simulink model "full_adder"  (R2015a)
settings: Solver=ode23t  StartTime=0.0  StopTime=4  RelTol=1e-3
libraries: fl_lib x281, nesl_utility x271, elec_lib x25
(part 1 of 4)
settings Model: Creator=tomas  LastModifiedBy=tomas

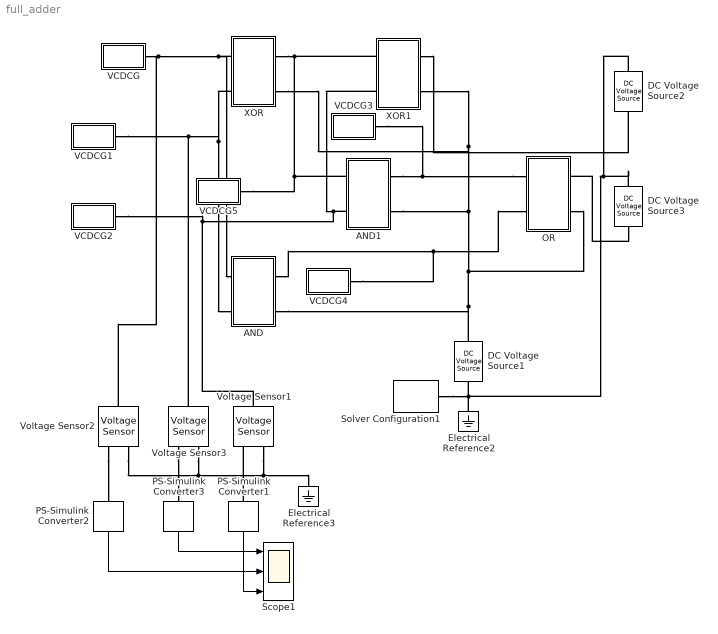
== system full_adder ==
  AND : Subsystem
  AND1 : Subsystem
  DC Voltage Source1 : fl_lib/Electrical/Electrical Sources/DC Voltage Source  v0=1 V
  DC Voltage Source2 : fl_lib/Electrical/Electrical Sources/DC Voltage Source  v0=1 V
  DC Voltage Source3 : fl_lib/Electrical/Electrical Sources/DC Voltage Source  v0=1 V
  Electrical Reference2 : fl_lib/Electrical/Electrical Elements/Electrical Reference
  Electrical Reference3 : fl_lib/Electrical/Electrical Elements/Electrical Reference
  OR : Subsystem
  PS-Simulink Converter1 : nesl_utility/PS-Simulink Converter  PhysicalDomain=network_engine_domain  SubClassName=ps_output  LeftPortType=input  RightPortType=output  PseudoPeriodic=off  Frequencies=[]  Unit=1  AffineConversion=off
  PS-Simulink Converter2 : nesl_utility/PS-Simulink Converter  PhysicalDomain=network_engine_domain  SubClassName=ps_output  LeftPortType=input  RightPortType=output  PseudoPeriodic=off  Frequencies=[]  Unit=1  AffineConversion=off
  PS-Simulink Converter3 : nesl_utility/PS-Simulink Converter  PhysicalDomain=network_engine_domain  SubClassName=ps_output  LeftPortType=input  RightPortType=output  PseudoPeriodic=off  Frequencies=[]  Unit=1  AffineConversion=off
  Scope1 : Scope  NumInputPorts=3
      settings: YMin=-10~-11~-5.5  YMax=0~0~-0.5
  Solver Configuration1 : nesl_utility/Solver Configuration  PhysicalDomain=network_engine_domain  SubClassName=solver  LeftPortType=input  RightPortType=generic  Accelerate=off  Tones=[]  Harmonics=[]  SimulateNoise=off  Profile=off  UseLocalSampling=off  EnableSwitchedLinearOptims=on  FrequencyDomain=off  UseCCode=off  RelTol=0.001  AbsTol=1e-06  MinStep=1e-09  ToWorkspace=off  RevertToSquareIcSolve=off  NumHomotopyIterations=100  DoDC=off  ResidualTolerance=1e-09  UseLocalSolver=off  LocalSolverChoice=NE_BACKWARD_EULER_ADVANCER  LocalSolverSampleTime=0.001  DoFixedCost=off  MaxNonlinIter=3  MaxModeIter=2  LinearAlgebra=Sparse  DelaysMemoryBudget=1024  AutomaticFiltering=on  FilteringTimeConstant=0.001
  VCDCG : Subsystem
  VCDCG1 : Subsystem
  VCDCG2 : Subsystem
  VCDCG3 : Subsystem
  VCDCG4 : Subsystem
  VCDCG5 : Subsystem
  Voltage Sensor1 : fl_lib/Electrical/Electrical Sensors/Voltage Sensor
  Voltage Sensor2 : fl_lib/Electrical/Electrical Sensors/Voltage Sensor
  Voltage Sensor3 : fl_lib/Electrical/Electrical Sensors/Voltage Sensor
  XOR : Subsystem
  XOR1 : Subsystem
  wires:
  PS-Simulink Converter3/1 -> Scope1/1
  PS-Simulink Converter2/1 -> Scope1/2
  PS-Simulink Converter1/1 -> Scope1/3
  connections:
  Electrical Reference2/LConn1 -- DC Voltage Source3/LConn1 -- DC Voltage Source2/LConn1 -- DC Voltage Source1/RConn1 -- Solver Configuration1/RConn1
  DC Voltage Source1/LConn1 -- AND1/RConn2 -- XOR1/RConn2 -- XOR/RConn2 -- OR/RConn2 -- AND/RConn2
  XOR/LConn2 -- VCDCG1/RConn1 -- Voltage Sensor3/LConn1 -- AND/LConn2
  XOR/LConn1 -- Voltage Sensor2/LConn1 -- VCDCG/RConn1 -- AND/LConn1
  XOR/RConn1 -- XOR1/LConn1 -- AND1/LConn1 -- VCDCG5/RConn1
  OR/LConn1 -- AND1/RConn1 -- VCDCG3/RConn1
  AND/RConn1 -- VCDCG4/RConn1 -- OR/LConn2
  VCDCG2/RConn1 -- Voltage Sensor1/LConn1 -- AND1/LConn2 -- XOR1/LConn2
  Voltage Sensor3/RConn2 -- Voltage Sensor2/RConn2 -- Voltage Sensor1/RConn2 -- Electrical Reference3/LConn1
  Voltage Sensor2/RConn1 -- PS-Simulink Converter2/LConn1
  Voltage Sensor3/RConn1 -- PS-Simulink Converter3/LConn1
  PS-Simulink Converter1/LConn1 -- Voltage Sensor1/RConn1
  DC Voltage Source3/RConn1 -- OR/RConn1
  XOR1/RConn1 -- DC Voltage Source2/RConn1

== system full_adder/AND ==
  DCM : Subsystem
  DCM1 : Subsystem
  DCM2 : Subsystem
  Electrical Reference : fl_lib/Electrical/Electrical Elements/Electrical Reference
  Electrical Reference1 : fl_lib/Electrical/Electrical Elements/Electrical Reference
  Out Terminal : Constant  Value=[1 0 0 0; 0 1 0 0; 0 0 1 0; 2 2 -1 -2; -4 -4 7 2]  VectorParams1D=off
  Resistor : elec_lib/Passive Devices/Resistor  R=16 kOhm  noise_mode=0  Tdevice=25 C  sample_time=0.001 s  repeatability=1  auto_seed=1456083514  user_seed=0
  Resistor1 : elec_lib/Passive Devices/Resistor  R=16 kOhm  noise_mode=0  Tdevice=25 C  sample_time=0.001 s  repeatability=1  auto_seed=3847689602  user_seed=0
  Terminal1 : Constant  Value=[0 -1 1 1; 1 0 0 0; 0 0 1 0; 1 0 0 0; 4 1 -3 -1]  VectorParams1D=off
  Terminal2 : Constant  Value=[-1 0 1 1; 0 1 0 0; 0 0 1 0; 0 1 0 0; 1 4 -3 -1]  VectorParams1D=off
  Voltage Sensor{,1..3} (4 alike) : fl_lib/Electrical/Electrical Sensors/Voltage Sensor
  v1 : PMIOPort  Port=1  Side=Left
  v2 : PMIOPort  Port=2  Side=Left
  vo : PMIOPort  Port=3  Side=Right
  vc : PMIOPort  Port=4  Side=Right
  wires:
  Terminal2/1 -> DCM1/1(m)
  Out Terminal/1 -> DCM2/1(m)
  Terminal1/1 -> DCM/1(m)
  connections:
  Voltage Sensor/LConn1 -- DCM/RConn2 -- Resistor/LConn1 -- v1/RConn1
  Voltage Sensor1/LConn1 -- DCM1/RConn2 -- Resistor1/LConn1 -- v2/RConn1
  DCM2/RConn1 -- Voltage Sensor1/RConn1 -- DCM1/RConn1 -- DCM/RConn1
  DCM2/LConn1 -- DCM1/LConn1 -- DCM/LConn1 -- Voltage Sensor/RConn1
  Voltage Sensor2/LConn1 -- DCM2/RConn2 -- Resistor/RConn1 -- Resistor1/RConn1 -- vo/RConn1
  Voltage Sensor2/RConn2 -- Voltage Sensor1/RConn2 -- Electrical Reference/LConn1 -- Voltage Sensor/RConn2
  DCM2/LConn2 -- Voltage Sensor2/RConn1 -- DCM1/LConn2 -- DCM/LConn2
  Voltage Sensor3/LConn1 -- vc/RConn1
  DCM2/LConn3 -- DCM1/LConn3 -- DCM/LConn3 -- Voltage Sensor3/RConn1
  Voltage Sensor3/RConn2 -- Electrical Reference1/LConn1

== system full_adder/AND1 ==
  DCM : Subsystem
  DCM1 : Subsystem
  DCM2 : Subsystem
  Electrical Reference : fl_lib/Electrical/Electrical Elements/Electrical Reference
  Electrical Reference1 : fl_lib/Electrical/Electrical Elements/Electrical Reference
  Out Terminal : Constant  Value=[1 0 0 0; 0 1 0 0; 0 0 1 0; 2 2 -1 -2; -4 -4 7 2]  VectorParams1D=off
  Resistor : elec_lib/Passive Devices/Resistor  R=16 kOhm  noise_mode=0  Tdevice=25 C  sample_time=0.001 s  repeatability=1  auto_seed=1903427766  user_seed=0
  Resistor1 : elec_lib/Passive Devices/Resistor  R=16 kOhm  noise_mode=0  Tdevice=25 C  sample_time=0.001 s  repeatability=1  auto_seed=400135898  user_seed=0
  Terminal1 : Constant  Value=[0 -1 1 1; 1 0 0 0; 0 0 1 0; 1 0 0 0; 4 1 -3 -1]  VectorParams1D=off
  Terminal2 : Constant  Value=[-1 0 1 1; 0 1 0 0; 0 0 1 0; 0 1 0 0; 1 4 -3 -1]  VectorParams1D=off
  Voltage Sensor{,1..3} (4 alike) : fl_lib/Electrical/Electrical Sensors/Voltage Sensor
  v1 : PMIOPort  Port=1  Side=Left
  v2 : PMIOPort  Port=2  Side=Left
  vo : PMIOPort  Port=3  Side=Right
  vc : PMIOPort  Port=4  Side=Right
  wires:
  Terminal2/1 -> DCM1/1(m)
  Out Terminal/1 -> DCM2/1(m)
  Terminal1/1 -> DCM/1(m)
  connections:
  Voltage Sensor/LConn1 -- Resistor/LConn1 -- v1/RConn1 -- DCM/RConn2
  Voltage Sensor1/LConn1 -- Resistor1/LConn1 -- v2/RConn1 -- DCM1/RConn2
  DCM1/RConn1 -- DCM/RConn1 -- Voltage Sensor1/RConn1 -- DCM2/RConn1
  DCM1/LConn1 -- DCM/LConn1 -- Voltage Sensor/RConn1 -- DCM2/LConn1
  Voltage Sensor2/LConn1 -- Resistor/RConn1 -- Resistor1/RConn1 -- vo/RConn1 -- DCM2/RConn2
  Voltage Sensor2/RConn2 -- Voltage Sensor1/RConn2 -- Electrical Reference/LConn1 -- Voltage Sensor/RConn2
  DCM1/LConn2 -- DCM/LConn2 -- Voltage Sensor2/RConn1 -- DCM2/LConn2
  Voltage Sensor3/LConn1 -- vc/RConn1
  DCM1/LConn3 -- DCM/LConn3 -- Voltage Sensor3/RConn1 -- DCM2/LConn3
  Voltage Sensor3/RConn2 -- Electrical Reference1/LConn1

== system full_adder/OR ==
  DCM : Subsystem
  DCM1 : Subsystem
  DCM2 : Subsystem
  Electrical Reference : fl_lib/Electrical/Electrical Elements/Electrical Reference
  Electrical Reference1 : fl_lib/Electrical/Electrical Elements/Electrical Reference
  Out Terminal : Constant  Value=[0 0 1 0; 2 2 -1 2; 1 0 0 0; 0 1 0 0; -4 -4 7 -2]  VectorParams1D=off  SampleTime=-1
  Resistor : elec_lib/Passive Devices/Resistor  R=16 kOhm  noise_mode=0  Tdevice=25 C  sample_time=0.001 s  repeatability=1  auto_seed=2834987259  user_seed=0
  Resistor1 : elec_lib/Passive Devices/Resistor  R=16 kOhm  noise_mode=0  Tdevice=25 C  sample_time=0.001 s  repeatability=1  auto_seed=2963978059  user_seed=0
  Terminal1 : Constant  Value=[0 0 1 0; 1 0 0 0; 0 -1 1 -1; 1 0 0 0; 4 1 -3 1]  VectorParams1D=off  SampleTime=-1
  Terminal2 : Constant  Value=[0 0 1 0; 0 1 0 0; -1 0 1 -1; 0 1 0 0; 1 4 -3 1 ]  VectorParams1D=off  SampleTime=-1
  Voltage Sensor{,1..3} (4 alike) : fl_lib/Electrical/Electrical Sensors/Voltage Sensor
  v1 : PMIOPort  Port=1  Side=Left
  v2 : PMIOPort  Port=2  Side=Left
  vo : PMIOPort  Port=3  Side=Right
  vc : PMIOPort  Port=4  Side=Right
  wires:
  Terminal2/1 -> DCM1/1(m)
  Out Terminal/1 -> DCM2/1(m)
  Terminal1/1 -> DCM/1(m)
  connections:
  Voltage Sensor/LConn1 -- DCM/RConn2 -- Resistor/LConn1 -- v1/RConn1
  Voltage Sensor1/LConn1 -- DCM1/RConn2 -- Resistor1/LConn1 -- v2/RConn1
  DCM2/RConn1 -- Voltage Sensor1/RConn1 -- DCM1/RConn1 -- DCM/RConn1
  DCM2/LConn1 -- DCM1/LConn1 -- DCM/LConn1 -- Voltage Sensor/RConn1
  Voltage Sensor2/LConn1 -- DCM2/RConn2 -- Resistor/RConn1 -- Resistor1/RConn1 -- vo/RConn1
  Voltage Sensor2/RConn2 -- Voltage Sensor1/RConn2 -- Electrical Reference/LConn1 -- Voltage Sensor/RConn2
  Voltage Sensor2/RConn1 -- DCM2/LConn2 -- DCM1/LConn2 -- DCM/LConn2
  Voltage Sensor3/LConn1 -- vc/RConn1
  DCM2/LConn3 -- DCM1/LConn3 -- DCM/LConn3 -- Voltage Sensor3/RConn1
  Voltage Sensor3/RConn2 -- Electrical Reference1/LConn1

== system full_adder/VCDCG ==
  Controlled Current Source : fl_lib/Electrical/Electrical Sources/Controlled Current Source
  Electrical Reference1 : fl_lib/Electrical/Electrical Elements/Electrical Reference
  Integrator : Integrator  InitialCondition=.001*rand()-.005  LimitOutput=on  UpperSaturationLimit=.2  LowerSaturationLimit=-.2
  MATLAB Function : MATLAB Function  TreatAsAtomicUnit=on
  PS-Simulink Converter : nesl_utility/PS-Simulink Converter  PhysicalDomain=network_engine_domain  SubClassName=ps_output  LeftPortType=input  RightPortType=output  PseudoPeriodic=off  Frequencies=[]  Unit=1  AffineConversion=off
  Simulink-PS Converter : nesl_utility/Simulink-PS Converter  PhysicalDomain=network_engine_domain  SubClassName=ps_input  LeftPortType=input  RightPortType=output  PseudoPeriodic=off  Frequencies=[]  NoiseDistribution=none  NoiseParameters=[]  Unit=1  AffineConversion=off  InputFiltering=off  SimscapeFilterOrder=1  InputFilterTimeConstant=0.001  UdotUserProvided=1
  Voltage Sensor : fl_lib/Electrical/Electrical Sensors/Voltage Sensor
  Out : PMIOPort  Port=1  Side=Right
  wires:
  Integrator/1 -> Simulink-PS Converter/1
  MATLAB Function/1(y) -> Integrator/1
  PS-Simulink Converter/1 -> MATLAB Function/1(u)
  connections:
  Voltage Sensor/RConn2 -- Controlled Current Source/RConn2 -- Electrical Reference1/LConn1
  Voltage Sensor/LConn1 -- Controlled Current Source/LConn1 -- Out/RConn1
  Voltage Sensor/RConn1 -- PS-Simulink Converter/LConn1
  Simulink-PS Converter/RConn1 -- Controlled Current Source/RConn1

== system full_adder/VCDCG1 ==
  Controlled Current Source : fl_lib/Electrical/Electrical Sources/Controlled Current Source
  Electrical Reference1 : fl_lib/Electrical/Electrical Elements/Electrical Reference
  Integrator : Integrator  InitialCondition=.001*rand()-.005  LimitOutput=on  UpperSaturationLimit=.2  LowerSaturationLimit=-.2
  MATLAB Function : MATLAB Function  TreatAsAtomicUnit=on
  PS-Simulink Converter : nesl_utility/PS-Simulink Converter  PhysicalDomain=network_engine_domain  SubClassName=ps_output  LeftPortType=input  RightPortType=output  PseudoPeriodic=off  Frequencies=[]  Unit=1  AffineConversion=off
  Simulink-PS Converter : nesl_utility/Simulink-PS Converter  PhysicalDomain=network_engine_domain  SubClassName=ps_input  LeftPortType=input  RightPortType=output  PseudoPeriodic=off  Frequencies=[]  NoiseDistribution=none  NoiseParameters=[]  Unit=1  AffineConversion=off  InputFiltering=off  SimscapeFilterOrder=1  InputFilterTimeConstant=0.001  UdotUserProvided=1
  Voltage Sensor : fl_lib/Electrical/Electrical Sensors/Voltage Sensor
  Out : PMIOPort  Port=1  Side=Right
  wires:
  Integrator/1 -> Simulink-PS Converter/1
  MATLAB Function/1(y) -> Integrator/1
  PS-Simulink Converter/1 -> MATLAB Function/1(u)
  connections:
  Electrical Reference1/LConn1 -- Voltage Sensor/RConn2 -- Controlled Current Source/RConn2
  Out/RConn1 -- Voltage Sensor/LConn1 -- Controlled Current Source/LConn1
  Voltage Sensor/RConn1 -- PS-Simulink Converter/LConn1
  Simulink-PS Converter/RConn1 -- Controlled Current Source/RConn1

== system full_adder/VCDCG2 ==
  Controlled Current Source : fl_lib/Electrical/Electrical Sources/Controlled Current Source
  Electrical Reference1 : fl_lib/Electrical/Electrical Elements/Electrical Reference
  Integrator : Integrator  InitialCondition=.001*rand()-.005  LimitOutput=on  UpperSaturationLimit=.2  LowerSaturationLimit=-.2
  MATLAB Function : MATLAB Function  TreatAsAtomicUnit=on
  PS-Simulink Converter : nesl_utility/PS-Simulink Converter  PhysicalDomain=network_engine_domain  SubClassName=ps_output  LeftPortType=input  RightPortType=output  PseudoPeriodic=off  Frequencies=[]  Unit=1  AffineConversion=off
  Simulink-PS Converter : nesl_utility/Simulink-PS Converter  PhysicalDomain=network_engine_domain  SubClassName=ps_input  LeftPortType=input  RightPortType=output  PseudoPeriodic=off  Frequencies=[]  NoiseDistribution=none  NoiseParameters=[]  Unit=1  AffineConversion=off  InputFiltering=off  SimscapeFilterOrder=1  InputFilterTimeConstant=0.001  UdotUserProvided=1
  Voltage Sensor : fl_lib/Electrical/Electrical Sensors/Voltage Sensor
  Out : PMIOPort  Port=1  Side=Right
  wires:
  Integrator/1 -> Simulink-PS Converter/1
  MATLAB Function/1(y) -> Integrator/1
  PS-Simulink Converter/1 -> MATLAB Function/1(u)
  connections:
  Electrical Reference1/LConn1 -- Voltage Sensor/RConn2 -- Controlled Current Source/RConn2
  Out/RConn1 -- Voltage Sensor/LConn1 -- Controlled Current Source/LConn1
  Voltage Sensor/RConn1 -- PS-Simulink Converter/LConn1
  Simulink-PS Converter/RConn1 -- Controlled Current Source/RConn1

== system full_adder/VCDCG3 ==
  Controlled Current Source : fl_lib/Electrical/Electrical Sources/Controlled Current Source
  Electrical Reference1 : fl_lib/Electrical/Electrical Elements/Electrical Reference
  Integrator : Integrator  InitialCondition=.001*rand()-.005  LimitOutput=on  UpperSaturationLimit=.2  LowerSaturationLimit=-.2
  MATLAB Function : MATLAB Function  TreatAsAtomicUnit=on
  PS-Simulink Converter : nesl_utility/PS-Simulink Converter  PhysicalDomain=network_engine_domain  SubClassName=ps_output  LeftPortType=input  RightPortType=output  PseudoPeriodic=off  Frequencies=[]  Unit=1  AffineConversion=off
  Simulink-PS Converter : nesl_utility/Simulink-PS Converter  PhysicalDomain=network_engine_domain  SubClassName=ps_input  LeftPortType=input  RightPortType=output  PseudoPeriodic=off  Frequencies=[]  NoiseDistribution=none  NoiseParameters=[]  Unit=1  AffineConversion=off  InputFiltering=off  SimscapeFilterOrder=1  InputFilterTimeConstant=0.001  UdotUserProvided=1
  Voltage Sensor : fl_lib/Electrical/Electrical Sensors/Voltage Sensor
  Out : PMIOPort  Port=1  Side=Right
  wires:
  Integrator/1 -> Simulink-PS Converter/1
  MATLAB Function/1(y) -> Integrator/1
  PS-Simulink Converter/1 -> MATLAB Function/1(u)
  connections:
  Electrical Reference1/LConn1 -- Voltage Sensor/RConn2 -- Controlled Current Source/RConn2
  Out/RConn1 -- Voltage Sensor/LConn1 -- Controlled Current Source/LConn1
  Voltage Sensor/RConn1 -- PS-Simulink Converter/LConn1
  Simulink-PS Converter/RConn1 -- Controlled Current Source/RConn1

== system full_adder/VCDCG4 ==
  Controlled Current Source : fl_lib/Electrical/Electrical Sources/Controlled Current Source
  Electrical Reference1 : fl_lib/Electrical/Electrical Elements/Electrical Reference
  Integrator : Integrator  InitialCondition=.001*rand()-.005  LimitOutput=on  UpperSaturationLimit=.2  LowerSaturationLimit=-.2
  MATLAB Function : MATLAB Function  TreatAsAtomicUnit=on
  PS-Simulink Converter : nesl_utility/PS-Simulink Converter  PhysicalDomain=network_engine_domain  SubClassName=ps_output  LeftPortType=input  RightPortType=output  PseudoPeriodic=off  Frequencies=[]  Unit=1  AffineConversion=off
  Simulink-PS Converter : nesl_utility/Simulink-PS Converter  PhysicalDomain=network_engine_domain  SubClassName=ps_input  LeftPortType=input  RightPortType=output  PseudoPeriodic=off  Frequencies=[]  NoiseDistribution=none  NoiseParameters=[]  Unit=1  AffineConversion=off  InputFiltering=off  SimscapeFilterOrder=1  InputFilterTimeConstant=0.001  UdotUserProvided=1
  Voltage Sensor : fl_lib/Electrical/Electrical Sensors/Voltage Sensor
  Out : PMIOPort  Port=1  Side=Right
  wires:
  Integrator/1 -> Simulink-PS Converter/1
  MATLAB Function/1(y) -> Integrator/1
  PS-Simulink Converter/1 -> MATLAB Function/1(u)
  connections:
  Electrical Reference1/LConn1 -- Voltage Sensor/RConn2 -- Controlled Current Source/RConn2
  Out/RConn1 -- Voltage Sensor/LConn1 -- Controlled Current Source/LConn1
  Voltage Sensor/RConn1 -- PS-Simulink Converter/LConn1
  Simulink-PS Converter/RConn1 -- Controlled Current Source/RConn1

== system full_adder/VCDCG5 ==
  Controlled Current Source : fl_lib/Electrical/Electrical Sources/Controlled Current Source
  Electrical Reference1 : fl_lib/Electrical/Electrical Elements/Electrical Reference
  Integrator : Integrator  InitialCondition=.001*rand()-.005  LimitOutput=on  UpperSaturationLimit=.2  LowerSaturationLimit=-.2
  MATLAB Function : MATLAB Function  TreatAsAtomicUnit=on
  PS-Simulink Converter : nesl_utility/PS-Simulink Converter  PhysicalDomain=network_engine_domain  SubClassName=ps_output  LeftPortType=input  RightPortType=output  PseudoPeriodic=off  Frequencies=[]  Unit=1  AffineConversion=off
  Simulink-PS Converter : nesl_utility/Simulink-PS Converter  PhysicalDomain=network_engine_domain  SubClassName=ps_input  LeftPortType=input  RightPortType=output  PseudoPeriodic=off  Frequencies=[]  NoiseDistribution=none  NoiseParameters=[]  Unit=1  AffineConversion=off  InputFiltering=off  SimscapeFilterOrder=1  InputFilterTimeConstant=0.001  UdotUserProvided=1
  Voltage Sensor : fl_lib/Electrical/Electrical Sensors/Voltage Sensor
  Out : PMIOPort  Port=1  Side=Right
  wires:
  Integrator/1 -> Simulink-PS Converter/1
  MATLAB Function/1(y) -> Integrator/1
  PS-Simulink Converter/1 -> MATLAB Function/1(u)
  connections:
  Electrical Reference1/LConn1 -- Voltage Sensor/RConn2 -- Controlled Current Source/RConn2
  Out/RConn1 -- Voltage Sensor/LConn1 -- Controlled Current Source/LConn1
  Voltage Sensor/RConn1 -- PS-Simulink Converter/LConn1
  Simulink-PS Converter/RConn1 -- Controlled Current Source/RConn1

== system full_adder/XOR ==
  DCM : Subsystem
  DCM1 : Subsystem
  DCM2 : Subsystem
  Electrical Reference : fl_lib/Electrical/Electrical Elements/Electrical Reference
  Electrical Reference1 : fl_lib/Electrical/Electrical Elements/Electrical Reference
  Out Terminal : Constant  Value=[-1 -1 0 1; 1 1 0 1; -1 1 0 -1; 1 -1 0 -1; -1 -1 7 0]  VectorParams1D=off
  Resistor : elec_lib/Passive Devices/Resistor  R=26 kOhm  noise_mode=0  Tdevice=25 C  sample_time=0.001 s  repeatability=1  auto_seed=3482499289  user_seed=0
  Resistor1 : elec_lib/Passive Devices/Resistor  R=26 kOhm  noise_mode=0  Tdevice=25 C  sample_time=0.001 s  repeatability=1  auto_seed=3989505789  user_seed=0
  Terminal1 : Constant  Value=[0 -1 -1 1; 0 1 1 1; 0 -1 1 -1; 0 1 -1 -1; 6 0 -1 0]  VectorParams1D=off
  Terminal2 : Constant  Value=[-1 0 -1 1; 1 0 1 1; -1 0 1 -1; 1 0 -1 -1; 0 6 -1 0]  VectorParams1D=off
  Voltage Sensor{,1..3} (4 alike) : fl_lib/Electrical/Electrical Sensors/Voltage Sensor
  v1 : PMIOPort  Port=1  Side=Left
  v2 : PMIOPort  Port=2  Side=Left
  vo : PMIOPort  Port=3  Side=Right
  vc : PMIOPort  Port=4  Side=Right
  wires:
  Terminal2/1 -> DCM1/1(m)
  Out Terminal/1 -> DCM2/1(m)
  Terminal1/1 -> DCM/1(m)
  connections:
  DCM/RConn2 -- Voltage Sensor/LConn1 -- Resistor/LConn1 -- v1/RConn1
  Voltage Sensor1/LConn1 -- DCM1/RConn2 -- Resistor1/LConn1 -- v2/RConn1
  DCM2/RConn1 -- Voltage Sensor1/RConn1 -- DCM1/RConn1 -- DCM/RConn1
  DCM2/LConn1 -- DCM1/LConn1 -- DCM/LConn1 -- Voltage Sensor/RConn1
  Voltage Sensor2/LConn1 -- DCM2/RConn2 -- Resistor/RConn1 -- Resistor1/RConn1 -- vo/RConn1
  Voltage Sensor2/RConn2 -- Voltage Sensor1/RConn2 -- Electrical Reference/LConn1 -- Voltage Sensor/RConn2
  DCM2/LConn2 -- Voltage Sensor2/RConn1 -- DCM1/LConn2 -- DCM/LConn2
  Voltage Sensor3/LConn1 -- vc/RConn1
  DCM2/LConn3 -- DCM1/LConn3 -- DCM/LConn3 -- Voltage Sensor3/RConn1
  Voltage Sensor3/RConn2 -- Electrical Reference1/LConn1

== system full_adder/XOR1 ==
  DCM : Subsystem
  DCM1 : Subsystem
  DCM2 : Subsystem
  Electrical Reference : fl_lib/Electrical/Electrical Elements/Electrical Reference
  Electrical Reference1 : fl_lib/Electrical/Electrical Elements/Electrical Reference
  Out Terminal : Constant  Value=[-1 -1 0 1; 1 1 0 1; -1 1 0 -1; 1 -1 0 -1; -1 -1 7 0]  VectorParams1D=off
  Resistor : elec_lib/Passive Devices/Resistor  R=26 kOhm  noise_mode=0  Tdevice=25 C  sample_time=0.001 s  repeatability=1  auto_seed=311627844  user_seed=0
  Resistor1 : elec_lib/Passive Devices/Resistor  R=26 kOhm  noise_mode=0  Tdevice=25 C  sample_time=0.001 s  repeatability=1  auto_seed=2729173630  user_seed=0
  Terminal1 : Constant  Value=[0 -1 -1 1; 0 1 1 1; 0 -1 1 -1; 0 1 -1 -1; 6 0 -1 0]  VectorParams1D=off
  Terminal2 : Constant  Value=[-1 0 -1 1; 1 0 1 1; -1 0 1 -1; 1 0 -1 -1; 0 6 -1 0]  VectorParams1D=off
  Voltage Sensor{,1..3} (4 alike) : fl_lib/Electrical/Electrical Sensors/Voltage Sensor
  v1 : PMIOPort  Port=1  Side=Left
  v2 : PMIOPort  Port=2  Side=Left
  vo : PMIOPort  Port=3  Side=Right
  vc : PMIOPort  Port=4  Side=Right
  wires:
  Terminal2/1 -> DCM1/1(m)
  Out Terminal/1 -> DCM2/1(m)
  Terminal1/1 -> DCM/1(m)
  connections:
  DCM/RConn2 -- Voltage Sensor/LConn1 -- Resistor/LConn1 -- v1/RConn1
  Voltage Sensor1/LConn1 -- Resistor1/LConn1 -- v2/RConn1 -- DCM1/RConn2
  DCM1/RConn1 -- DCM/RConn1 -- Voltage Sensor1/RConn1 -- DCM2/RConn1
  DCM1/LConn1 -- DCM/LConn1 -- Voltage Sensor/RConn1 -- DCM2/LConn1
  Voltage Sensor2/LConn1 -- Resistor/RConn1 -- Resistor1/RConn1 -- vo/RConn1 -- DCM2/RConn2
  Voltage Sensor2/RConn2 -- Voltage Sensor1/RConn2 -- Electrical Reference/LConn1 -- Voltage Sensor/RConn2
  DCM1/LConn2 -- DCM/LConn2 -- Voltage Sensor2/RConn1 -- DCM2/LConn2
  Voltage Sensor3/LConn1 -- vc/RConn1
  DCM1/LConn3 -- DCM/LConn3 -- Voltage Sensor3/RConn1 -- DCM2/LConn3
  Voltage Sensor3/RConn2 -- Electrical Reference1/LConn1

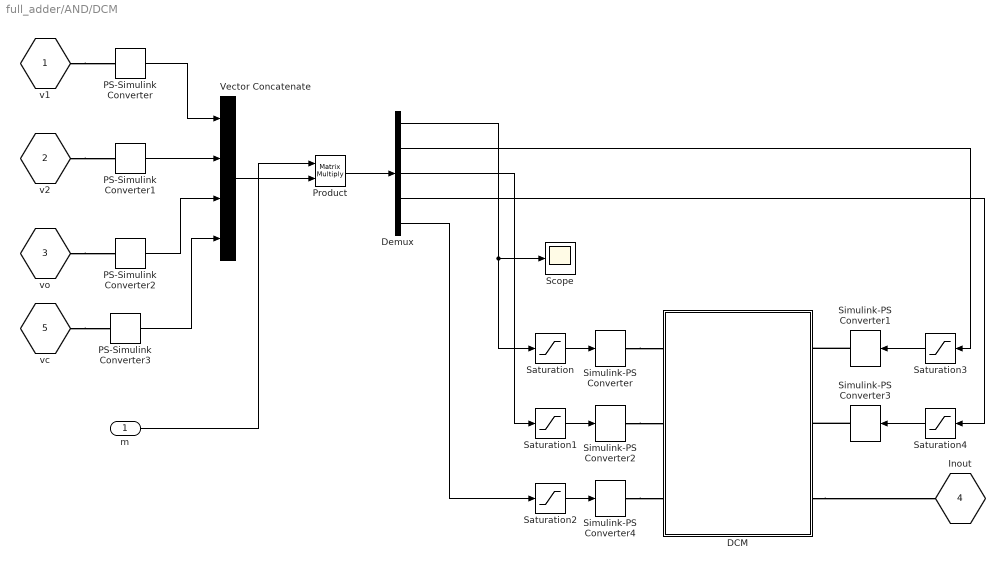
== system full_adder/AND/DCM ==
  m : Inport
  DCM : Subsystem
  Demux : Demux  Outputs=5
  PS-Simulink Converter{,1..3} (4 alike) : nesl_utility/PS-Simulink Converter  PhysicalDomain=network_engine_domain  SubClassName=ps_output  LeftPortType=input  RightPortType=output  PseudoPeriodic=off  Frequencies=[]  Unit=V  AffineConversion=off
  Product : Product  Multiplication=Matrix(*)
  Saturation{,1..4} (5 alike) : Saturate  UpperLimit=10  LowerLimit=-10
  Scope : Scope
      settings: YMin=-30  YMax=15  SaveName=ScopeData3
  Simulink-PS Converter{,1..4} (5 alike) : nesl_utility/Simulink-PS Converter  PhysicalDomain=network_engine_domain  SubClassName=ps_input  LeftPortType=input  RightPortType=output  PseudoPeriodic=off  Frequencies=[]  NoiseDistribution=none  NoiseParameters=[]  Unit=V  AffineConversion=off  InputFiltering=off  SimscapeFilterOrder=1  InputFilterTimeConstant=0.001  UdotUserProvided=1
  Vector Concatenate : Concatenate  NumInputs=4
  "v1 " : PMIOPort  Port=1  Side=Left
  v2 : PMIOPort  Port=2  Side=Right
  vo : PMIOPort  Port=3  Side=Left
  Inout : PMIOPort  Port=4  Side=Right
  vc : PMIOPort  Port=5  Side=Left
  wires:
  PS-Simulink Converter3/1 -> Vector Concatenate/4
  PS-Simulink Converter/1 -> Vector Concatenate/1
  PS-Simulink Converter2/1 -> Vector Concatenate/3
  PS-Simulink Converter1/1 -> Vector Concatenate/2
  Demux/1 -> Scope/1, Saturation/1
  m/1 -> Product/1
  Vector Concatenate/1 -> Product/2
  Product/1 -> Demux/1
  Saturation/1 -> Simulink-PS Converter/1
  Demux/3 -> Saturation1/1
  Saturation1/1 -> Simulink-PS Converter2/1
  Demux/5 -> Saturation2/1
  Saturation2/1 -> Simulink-PS Converter4/1
  Saturation3/1 -> Simulink-PS Converter1/1
  Demux/2 -> Saturation3/1
  Saturation4/1 -> Simulink-PS Converter3/1
  Demux/4 -> Saturation4/1
  connections:
  Simulink-PS Converter2/RConn1 -- DCM/LConn2
  DCM/RConn3 -- Inout/RConn1
  Simulink-PS Converter3/RConn1 -- DCM/RConn2
  vo/RConn1 -- PS-Simulink Converter2/LConn1
  Simulink-PS Converter4/RConn1 -- DCM/LConn3
  Simulink-PS Converter/RConn1 -- DCM/LConn1
  "v1 "/RConn1 -- PS-Simulink Converter/LConn1
  v2/RConn1 -- PS-Simulink Converter1/LConn1
  Simulink-PS Converter1/RConn1 -- DCM/RConn1
  vc/RConn1 -- PS-Simulink Converter3/LConn1

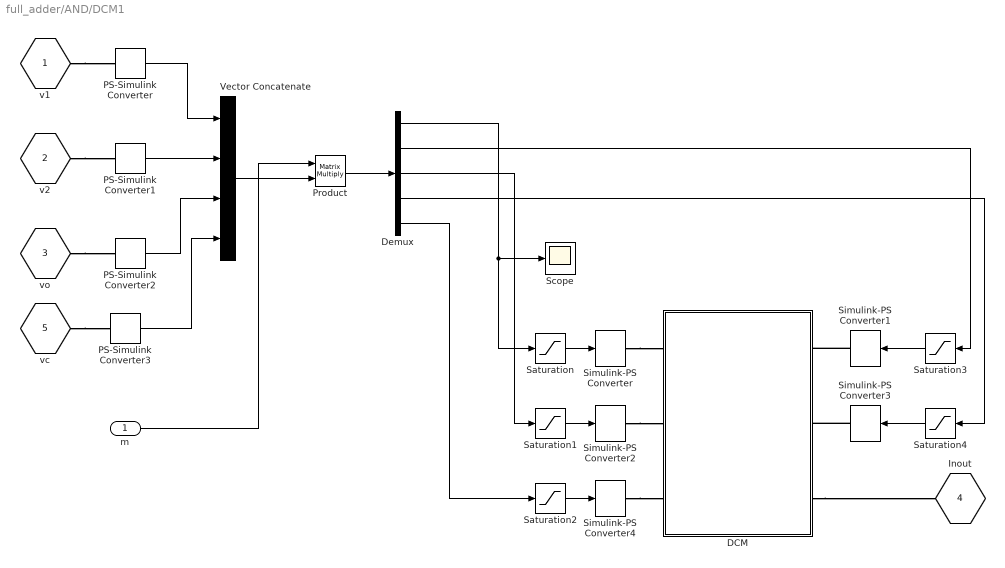
== system full_adder/AND/DCM1 ==
  m : Inport
  DCM : Subsystem
  Demux : Demux  Outputs=5
  PS-Simulink Converter{,1..3} (4 alike) : nesl_utility/PS-Simulink Converter  PhysicalDomain=network_engine_domain  SubClassName=ps_output  LeftPortType=input  RightPortType=output  PseudoPeriodic=off  Frequencies=[]  Unit=V  AffineConversion=off
  Product : Product  Multiplication=Matrix(*)
  Saturation{,1..4} (5 alike) : Saturate  UpperLimit=10  LowerLimit=-10
  Scope : Scope
      settings: YMin=-30  YMax=15  SaveName=ScopeData3
  Simulink-PS Converter{,1..4} (5 alike) : nesl_utility/Simulink-PS Converter  PhysicalDomain=network_engine_domain  SubClassName=ps_input  LeftPortType=input  RightPortType=output  PseudoPeriodic=off  Frequencies=[]  NoiseDistribution=none  NoiseParameters=[]  Unit=V  AffineConversion=off  InputFiltering=off  SimscapeFilterOrder=1  InputFilterTimeConstant=0.001  UdotUserProvided=1
  Vector Concatenate : Concatenate  NumInputs=4
  "v1 " : PMIOPort  Port=1  Side=Left
  v2 : PMIOPort  Port=2  Side=Right
  vo : PMIOPort  Port=3  Side=Left
  Inout : PMIOPort  Port=4  Side=Right
  vc : PMIOPort  Port=5  Side=Left
  wires:
  PS-Simulink Converter3/1 -> Vector Concatenate/4
  PS-Simulink Converter/1 -> Vector Concatenate/1
  PS-Simulink Converter2/1 -> Vector Concatenate/3
  PS-Simulink Converter1/1 -> Vector Concatenate/2
  Demux/1 -> Scope/1, Saturation/1
  m/1 -> Product/1
  Vector Concatenate/1 -> Product/2
  Product/1 -> Demux/1
  Saturation/1 -> Simulink-PS Converter/1
  Demux/3 -> Saturation1/1
  Saturation1/1 -> Simulink-PS Converter2/1
  Demux/5 -> Saturation2/1
  Saturation2/1 -> Simulink-PS Converter4/1
  Saturation3/1 -> Simulink-PS Converter1/1
  Demux/2 -> Saturation3/1
  Saturation4/1 -> Simulink-PS Converter3/1
  Demux/4 -> Saturation4/1
  connections:
  Simulink-PS Converter2/RConn1 -- DCM/LConn2
  DCM/RConn3 -- Inout/RConn1
  Simulink-PS Converter3/RConn1 -- DCM/RConn2
  vo/RConn1 -- PS-Simulink Converter2/LConn1
  Simulink-PS Converter4/RConn1 -- DCM/LConn3
  Simulink-PS Converter/RConn1 -- DCM/LConn1
  "v1 "/RConn1 -- PS-Simulink Converter/LConn1
  v2/RConn1 -- PS-Simulink Converter1/LConn1
  Simulink-PS Converter1/RConn1 -- DCM/RConn1
  vc/RConn1 -- PS-Simulink Converter3/LConn1

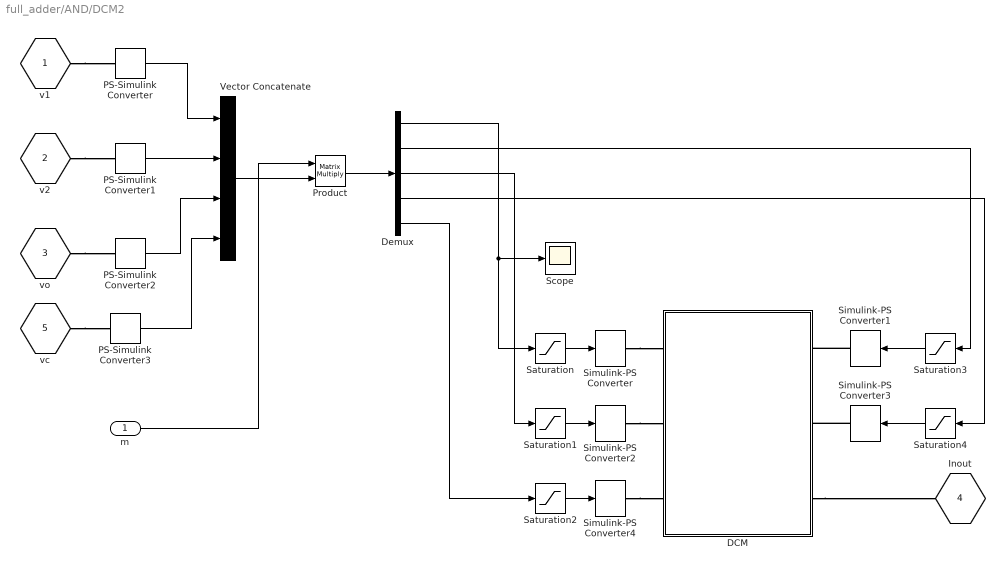
== system full_adder/AND/DCM2 ==
  m : Inport
  DCM : Subsystem
  Demux : Demux  Outputs=5
  PS-Simulink Converter{,1..3} (4 alike) : nesl_utility/PS-Simulink Converter  PhysicalDomain=network_engine_domain  SubClassName=ps_output  LeftPortType=input  RightPortType=output  PseudoPeriodic=off  Frequencies=[]  Unit=V  AffineConversion=off
  Product : Product  Multiplication=Matrix(*)
  Saturation{,1..4} (5 alike) : Saturate  UpperLimit=10  LowerLimit=-10
  Scope : Scope
      settings: YMin=-30  YMax=15  SaveName=ScopeData3
  Simulink-PS Converter{,1..4} (5 alike) : nesl_utility/Simulink-PS Converter  PhysicalDomain=network_engine_domain  SubClassName=ps_input  LeftPortType=input  RightPortType=output  PseudoPeriodic=off  Frequencies=[]  NoiseDistribution=none  NoiseParameters=[]  Unit=V  AffineConversion=off  InputFiltering=off  SimscapeFilterOrder=1  InputFilterTimeConstant=0.001  UdotUserProvided=1
  Vector Concatenate : Concatenate  NumInputs=4
  "v1 " : PMIOPort  Port=1  Side=Left
  v2 : PMIOPort  Port=2  Side=Right
  vo : PMIOPort  Port=3  Side=Left
  Inout : PMIOPort  Port=4  Side=Right
  vc : PMIOPort  Port=5  Side=Left
  wires:
  PS-Simulink Converter3/1 -> Vector Concatenate/4
  PS-Simulink Converter/1 -> Vector Concatenate/1
  PS-Simulink Converter2/1 -> Vector Concatenate/3
  PS-Simulink Converter1/1 -> Vector Concatenate/2
  Demux/1 -> Scope/1, Saturation/1
  m/1 -> Product/1
  Vector Concatenate/1 -> Product/2
  Product/1 -> Demux/1
  Saturation/1 -> Simulink-PS Converter/1
  Demux/3 -> Saturation1/1
  Saturation1/1 -> Simulink-PS Converter2/1
  Demux/5 -> Saturation2/1
  Saturation2/1 -> Simulink-PS Converter4/1
  Saturation3/1 -> Simulink-PS Converter1/1
  Demux/2 -> Saturation3/1
  Saturation4/1 -> Simulink-PS Converter3/1
  Demux/4 -> Saturation4/1
  connections:
  Simulink-PS Converter2/RConn1 -- DCM/LConn2
  DCM/RConn3 -- Inout/RConn1
  Simulink-PS Converter3/RConn1 -- DCM/RConn2
  vo/RConn1 -- PS-Simulink Converter2/LConn1
  Simulink-PS Converter4/RConn1 -- DCM/LConn3
  Simulink-PS Converter/RConn1 -- DCM/LConn1
  "v1 "/RConn1 -- PS-Simulink Converter/LConn1
  v2/RConn1 -- PS-Simulink Converter1/LConn1
  Simulink-PS Converter1/RConn1 -- DCM/RConn1
  vc/RConn1 -- PS-Simulink Converter3/LConn1

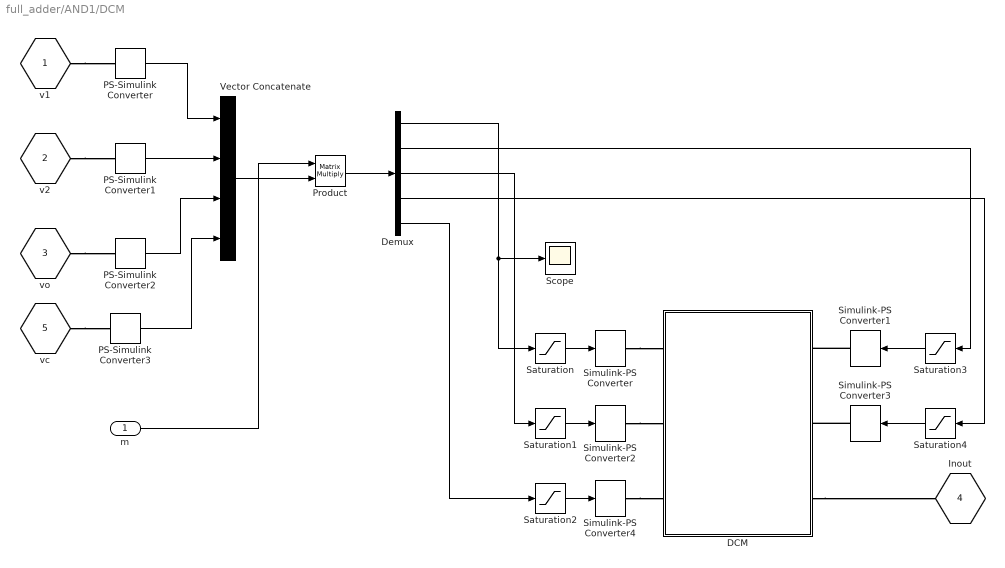
== system full_adder/AND1/DCM ==
  m : Inport
  DCM : Subsystem
  Demux : Demux  Outputs=5
  PS-Simulink Converter{,1..3} (4 alike) : nesl_utility/PS-Simulink Converter  PhysicalDomain=network_engine_domain  SubClassName=ps_output  LeftPortType=input  RightPortType=output  PseudoPeriodic=off  Frequencies=[]  Unit=V  AffineConversion=off
  Product : Product  Multiplication=Matrix(*)
  Saturation{,1..4} (5 alike) : Saturate  UpperLimit=10  LowerLimit=-10
  Scope : Scope
      settings: YMin=-30  YMax=15  SaveName=ScopeData3
  Simulink-PS Converter{,1..4} (5 alike) : nesl_utility/Simulink-PS Converter  PhysicalDomain=network_engine_domain  SubClassName=ps_input  LeftPortType=input  RightPortType=output  PseudoPeriodic=off  Frequencies=[]  NoiseDistribution=none  NoiseParameters=[]  Unit=V  AffineConversion=off  InputFiltering=off  SimscapeFilterOrder=1  InputFilterTimeConstant=0.001  UdotUserProvided=1
  Vector Concatenate : Concatenate  NumInputs=4
  "v1 " : PMIOPort  Port=1  Side=Left
  v2 : PMIOPort  Port=2  Side=Right
  vo : PMIOPort  Port=3  Side=Left
  Inout : PMIOPort  Port=4  Side=Right
  vc : PMIOPort  Port=5  Side=Left
  wires:
  PS-Simulink Converter3/1 -> Vector Concatenate/4
  PS-Simulink Converter/1 -> Vector Concatenate/1
  PS-Simulink Converter2/1 -> Vector Concatenate/3
  PS-Simulink Converter1/1 -> Vector Concatenate/2
  Demux/1 -> Scope/1, Saturation/1
  m/1 -> Product/1
  Vector Concatenate/1 -> Product/2
  Product/1 -> Demux/1
  Saturation/1 -> Simulink-PS Converter/1
  Demux/3 -> Saturation1/1
  Saturation1/1 -> Simulink-PS Converter2/1
  Demux/5 -> Saturation2/1
  Saturation2/1 -> Simulink-PS Converter4/1
  Saturation3/1 -> Simulink-PS Converter1/1
  Demux/2 -> Saturation3/1
  Saturation4/1 -> Simulink-PS Converter3/1
  Demux/4 -> Saturation4/1
  connections:
  Simulink-PS Converter2/RConn1 -- DCM/LConn2
  DCM/RConn3 -- Inout/RConn1
  Simulink-PS Converter3/RConn1 -- DCM/RConn2
  vo/RConn1 -- PS-Simulink Converter2/LConn1
  Simulink-PS Converter4/RConn1 -- DCM/LConn3
  Simulink-PS Converter/RConn1 -- DCM/LConn1
  "v1 "/RConn1 -- PS-Simulink Converter/LConn1
  v2/RConn1 -- PS-Simulink Converter1/LConn1
  Simulink-PS Converter1/RConn1 -- DCM/RConn1
  vc/RConn1 -- PS-Simulink Converter3/LConn1

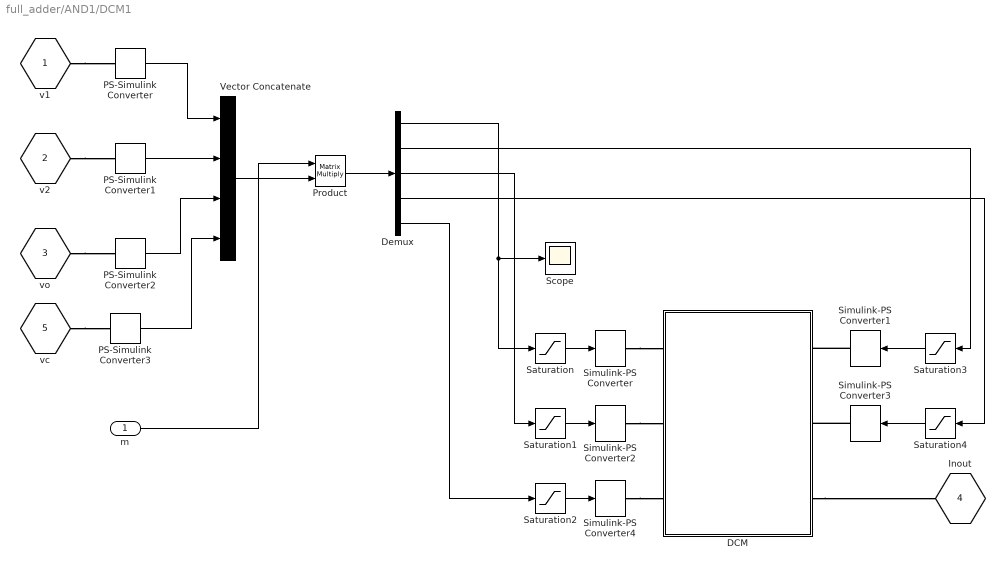
== system full_adder/AND1/DCM1 ==
  m : Inport
  DCM : Subsystem
  Demux : Demux  Outputs=5
  PS-Simulink Converter{,1..3} (4 alike) : nesl_utility/PS-Simulink Converter  PhysicalDomain=network_engine_domain  SubClassName=ps_output  LeftPortType=input  RightPortType=output  PseudoPeriodic=off  Frequencies=[]  Unit=V  AffineConversion=off
  Product : Product  Multiplication=Matrix(*)
  Saturation{,1..4} (5 alike) : Saturate  UpperLimit=10  LowerLimit=-10
  Scope : Scope
      settings: YMin=-30  YMax=15  SaveName=ScopeData3
  Simulink-PS Converter{,1..4} (5 alike) : nesl_utility/Simulink-PS Converter  PhysicalDomain=network_engine_domain  SubClassName=ps_input  LeftPortType=input  RightPortType=output  PseudoPeriodic=off  Frequencies=[]  NoiseDistribution=none  NoiseParameters=[]  Unit=V  AffineConversion=off  InputFiltering=off  SimscapeFilterOrder=1  InputFilterTimeConstant=0.001  UdotUserProvided=1
  Vector Concatenate : Concatenate  NumInputs=4
  "v1 " : PMIOPort  Port=1  Side=Left
  v2 : PMIOPort  Port=2  Side=Right
  vo : PMIOPort  Port=3  Side=Left
  Inout : PMIOPort  Port=4  Side=Right
  vc : PMIOPort  Port=5  Side=Left
  wires:
  PS-Simulink Converter3/1 -> Vector Concatenate/4
  PS-Simulink Converter/1 -> Vector Concatenate/1
  PS-Simulink Converter2/1 -> Vector Concatenate/3
  PS-Simulink Converter1/1 -> Vector Concatenate/2
  Demux/1 -> Scope/1, Saturation/1
  m/1 -> Product/1
  Vector Concatenate/1 -> Product/2
  Product/1 -> Demux/1
  Saturation/1 -> Simulink-PS Converter/1
  Demux/3 -> Saturation1/1
  Saturation1/1 -> Simulink-PS Converter2/1
  Demux/5 -> Saturation2/1
  Saturation2/1 -> Simulink-PS Converter4/1
  Saturation3/1 -> Simulink-PS Converter1/1
  Demux/2 -> Saturation3/1
  Saturation4/1 -> Simulink-PS Converter3/1
  Demux/4 -> Saturation4/1
  connections:
  Simulink-PS Converter2/RConn1 -- DCM/LConn2
  DCM/RConn3 -- Inout/RConn1
  Simulink-PS Converter3/RConn1 -- DCM/RConn2
  vo/RConn1 -- PS-Simulink Converter2/LConn1
  Simulink-PS Converter4/RConn1 -- DCM/LConn3
  Simulink-PS Converter/RConn1 -- DCM/LConn1
  "v1 "/RConn1 -- PS-Simulink Converter/LConn1
  v2/RConn1 -- PS-Simulink Converter1/LConn1
  Simulink-PS Converter1/RConn1 -- DCM/RConn1
  vc/RConn1 -- PS-Simulink Converter3/LConn1

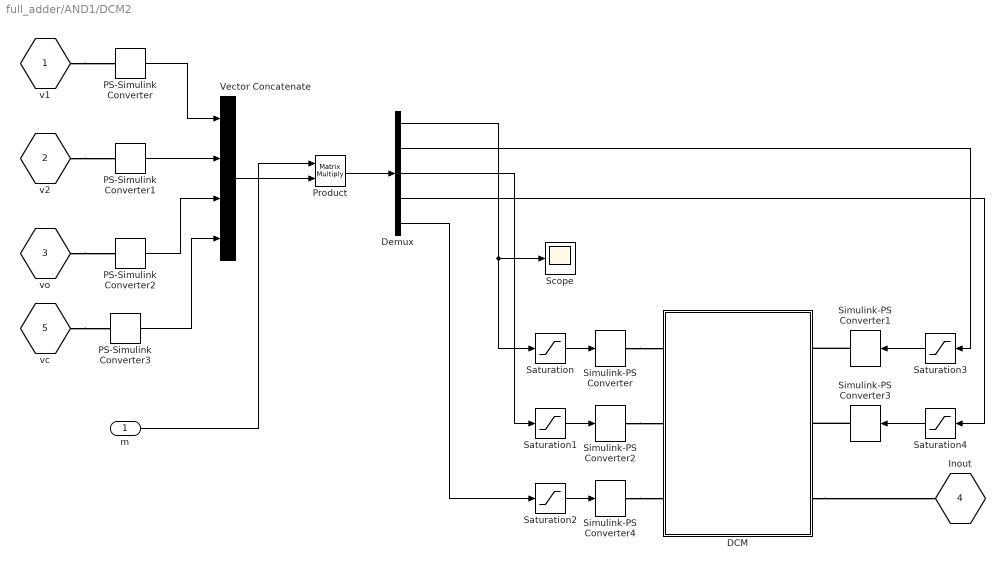
== system full_adder/AND1/DCM2 ==
  m : Inport
  DCM : Subsystem
  Demux : Demux  Outputs=5
  PS-Simulink Converter{,1..3} (4 alike) : nesl_utility/PS-Simulink Converter  PhysicalDomain=network_engine_domain  SubClassName=ps_output  LeftPortType=input  RightPortType=output  PseudoPeriodic=off  Frequencies=[]  Unit=V  AffineConversion=off
  Product : Product  Multiplication=Matrix(*)
  Saturation{,1..4} (5 alike) : Saturate  UpperLimit=10  LowerLimit=-10
  Scope : Scope
      settings: YMin=-30  YMax=15  SaveName=ScopeData3
  Simulink-PS Converter{,1..4} (5 alike) : nesl_utility/Simulink-PS Converter  PhysicalDomain=network_engine_domain  SubClassName=ps_input  LeftPortType=input  RightPortType=output  PseudoPeriodic=off  Frequencies=[]  NoiseDistribution=none  NoiseParameters=[]  Unit=V  AffineConversion=off  InputFiltering=off  SimscapeFilterOrder=1  InputFilterTimeConstant=0.001  UdotUserProvided=1
  Vector Concatenate : Concatenate  NumInputs=4
  "v1 " : PMIOPort  Port=1  Side=Left
  v2 : PMIOPort  Port=2  Side=Right
  vo : PMIOPort  Port=3  Side=Left
  Inout : PMIOPort  Port=4  Side=Right
  vc : PMIOPort  Port=5  Side=Left
  wires:
  PS-Simulink Converter3/1 -> Vector Concatenate/4
  PS-Simulink Converter/1 -> Vector Concatenate/1
  PS-Simulink Converter2/1 -> Vector Concatenate/3
  PS-Simulink Converter1/1 -> Vector Concatenate/2
  Demux/1 -> Scope/1, Saturation/1
  m/1 -> Product/1
  Vector Concatenate/1 -> Product/2
  Product/1 -> Demux/1
  Saturation/1 -> Simulink-PS Converter/1
  Demux/3 -> Saturation1/1
  Saturation1/1 -> Simulink-PS Converter2/1
  Demux/5 -> Saturation2/1
  Saturation2/1 -> Simulink-PS Converter4/1
  Saturation3/1 -> Simulink-PS Converter1/1
  Demux/2 -> Saturation3/1
  Saturation4/1 -> Simulink-PS Converter3/1
  Demux/4 -> Saturation4/1
  connections:
  Simulink-PS Converter2/RConn1 -- DCM/LConn2
  DCM/RConn3 -- Inout/RConn1
  Simulink-PS Converter3/RConn1 -- DCM/RConn2
  vo/RConn1 -- PS-Simulink Converter2/LConn1
  Simulink-PS Converter4/RConn1 -- DCM/LConn3
  Simulink-PS Converter/RConn1 -- DCM/LConn1
  "v1 "/RConn1 -- PS-Simulink Converter/LConn1
  v2/RConn1 -- PS-Simulink Converter1/LConn1
  Simulink-PS Converter1/RConn1 -- DCM/RConn1
  vc/RConn1 -- PS-Simulink Converter3/LConn1

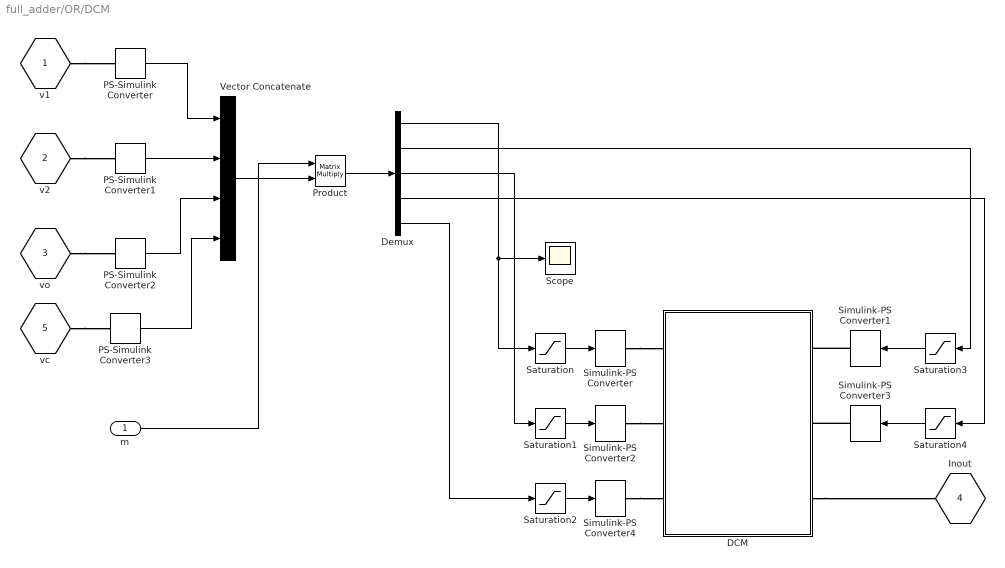
== system full_adder/OR/DCM ==
  m : Inport
  DCM : Subsystem
  Demux : Demux  Outputs=5
  PS-Simulink Converter{,1..3} (4 alike) : nesl_utility/PS-Simulink Converter  PhysicalDomain=network_engine_domain  SubClassName=ps_output  LeftPortType=input  RightPortType=output  PseudoPeriodic=off  Frequencies=[]  Unit=V  AffineConversion=off
  Product : Product  Multiplication=Matrix(*)
  Saturation{,1..4} (5 alike) : Saturate  UpperLimit=10  LowerLimit=-10
  Scope : Scope
      settings: YMin=-30  YMax=15  SaveName=ScopeData3
  Simulink-PS Converter{,1..4} (5 alike) : nesl_utility/Simulink-PS Converter  PhysicalDomain=network_engine_domain  SubClassName=ps_input  LeftPortType=input  RightPortType=output  PseudoPeriodic=off  Frequencies=[]  NoiseDistribution=none  NoiseParameters=[]  Unit=V  AffineConversion=off  InputFiltering=off  SimscapeFilterOrder=1  InputFilterTimeConstant=0.001  UdotUserProvided=1
  Vector Concatenate : Concatenate  NumInputs=4
  "v1 " : PMIOPort  Port=1  Side=Left
  v2 : PMIOPort  Port=2  Side=Right
  vo : PMIOPort  Port=3  Side=Left
  Inout : PMIOPort  Port=4  Side=Right
  vc : PMIOPort  Port=5  Side=Left
  wires:
  PS-Simulink Converter3/1 -> Vector Concatenate/4
  PS-Simulink Converter/1 -> Vector Concatenate/1
  PS-Simulink Converter2/1 -> Vector Concatenate/3
  PS-Simulink Converter1/1 -> Vector Concatenate/2
  Demux/1 -> Scope/1, Saturation/1
  m/1 -> Product/1
  Vector Concatenate/1 -> Product/2
  Product/1 -> Demux/1
  Saturation/1 -> Simulink-PS Converter/1
  Demux/3 -> Saturation1/1
  Saturation1/1 -> Simulink-PS Converter2/1
  Demux/5 -> Saturation2/1
  Saturation2/1 -> Simulink-PS Converter4/1
  Saturation3/1 -> Simulink-PS Converter1/1
  Demux/2 -> Saturation3/1
  Saturation4/1 -> Simulink-PS Converter3/1
  Demux/4 -> Saturation4/1
  connections:
  Simulink-PS Converter2/RConn1 -- DCM/LConn2
  DCM/RConn3 -- Inout/RConn1
  Simulink-PS Converter3/RConn1 -- DCM/RConn2
  vo/RConn1 -- PS-Simulink Converter2/LConn1
  Simulink-PS Converter4/RConn1 -- DCM/LConn3
  Simulink-PS Converter/RConn1 -- DCM/LConn1
  "v1 "/RConn1 -- PS-Simulink Converter/LConn1
  v2/RConn1 -- PS-Simulink Converter1/LConn1
  Simulink-PS Converter1/RConn1 -- DCM/RConn1
  vc/RConn1 -- PS-Simulink Converter3/LConn1

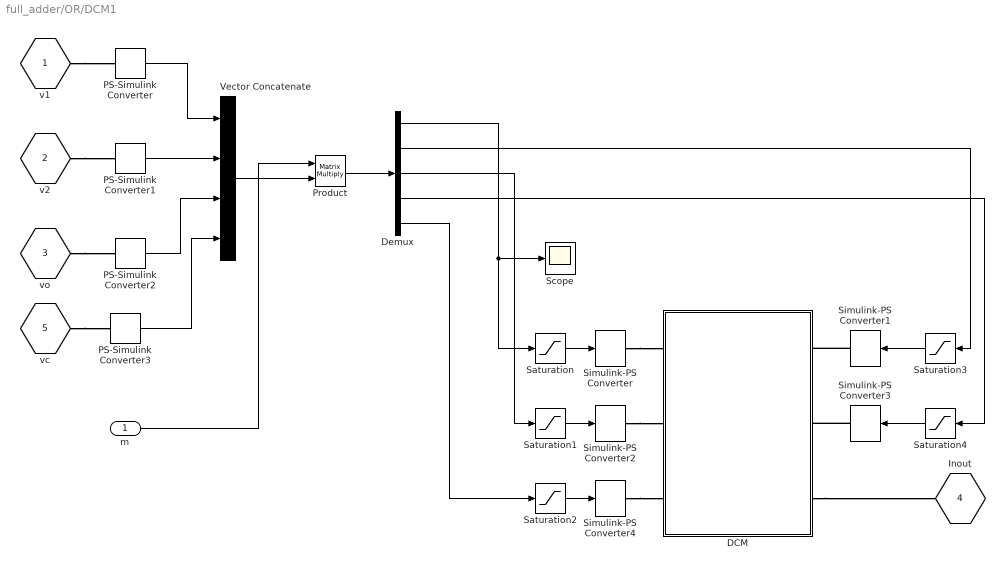
== system full_adder/OR/DCM1 ==
  m : Inport
  DCM : Subsystem
  Demux : Demux  Outputs=5
  PS-Simulink Converter{,1..3} (4 alike) : nesl_utility/PS-Simulink Converter  PhysicalDomain=network_engine_domain  SubClassName=ps_output  LeftPortType=input  RightPortType=output  PseudoPeriodic=off  Frequencies=[]  Unit=V  AffineConversion=off
  Product : Product  Multiplication=Matrix(*)
  Saturation{,1..4} (5 alike) : Saturate  UpperLimit=10  LowerLimit=-10
  Scope : Scope
      settings: YMin=-30  YMax=15  SaveName=ScopeData3
  Simulink-PS Converter{,1..4} (5 alike) : nesl_utility/Simulink-PS Converter  PhysicalDomain=network_engine_domain  SubClassName=ps_input  LeftPortType=input  RightPortType=output  PseudoPeriodic=off  Frequencies=[]  NoiseDistribution=none  NoiseParameters=[]  Unit=V  AffineConversion=off  InputFiltering=off  SimscapeFilterOrder=1  InputFilterTimeConstant=0.001  UdotUserProvided=1
  Vector Concatenate : Concatenate  NumInputs=4
  "v1 " : PMIOPort  Port=1  Side=Left
  v2 : PMIOPort  Port=2  Side=Right
  vo : PMIOPort  Port=3  Side=Left
  Inout : PMIOPort  Port=4  Side=Right
  vc : PMIOPort  Port=5  Side=Left
  wires:
  PS-Simulink Converter3/1 -> Vector Concatenate/4
  PS-Simulink Converter/1 -> Vector Concatenate/1
  PS-Simulink Converter2/1 -> Vector Concatenate/3
  PS-Simulink Converter1/1 -> Vector Concatenate/2
  Demux/1 -> Scope/1, Saturation/1
  m/1 -> Product/1
  Vector Concatenate/1 -> Product/2
  Product/1 -> Demux/1
  Saturation/1 -> Simulink-PS Converter/1
  Demux/3 -> Saturation1/1
  Saturation1/1 -> Simulink-PS Converter2/1
  Demux/5 -> Saturation2/1
  Saturation2/1 -> Simulink-PS Converter4/1
  Saturation3/1 -> Simulink-PS Converter1/1
  Demux/2 -> Saturation3/1
  Saturation4/1 -> Simulink-PS Converter3/1
  Demux/4 -> Saturation4/1
  connections:
  Simulink-PS Converter2/RConn1 -- DCM/LConn2
  DCM/RConn3 -- Inout/RConn1
  Simulink-PS Converter3/RConn1 -- DCM/RConn2
  vo/RConn1 -- PS-Simulink Converter2/LConn1
  Simulink-PS Converter4/RConn1 -- DCM/LConn3
  Simulink-PS Converter/RConn1 -- DCM/LConn1
  "v1 "/RConn1 -- PS-Simulink Converter/LConn1
  v2/RConn1 -- PS-Simulink Converter1/LConn1
  Simulink-PS Converter1/RConn1 -- DCM/RConn1
  vc/RConn1 -- PS-Simulink Converter3/LConn1

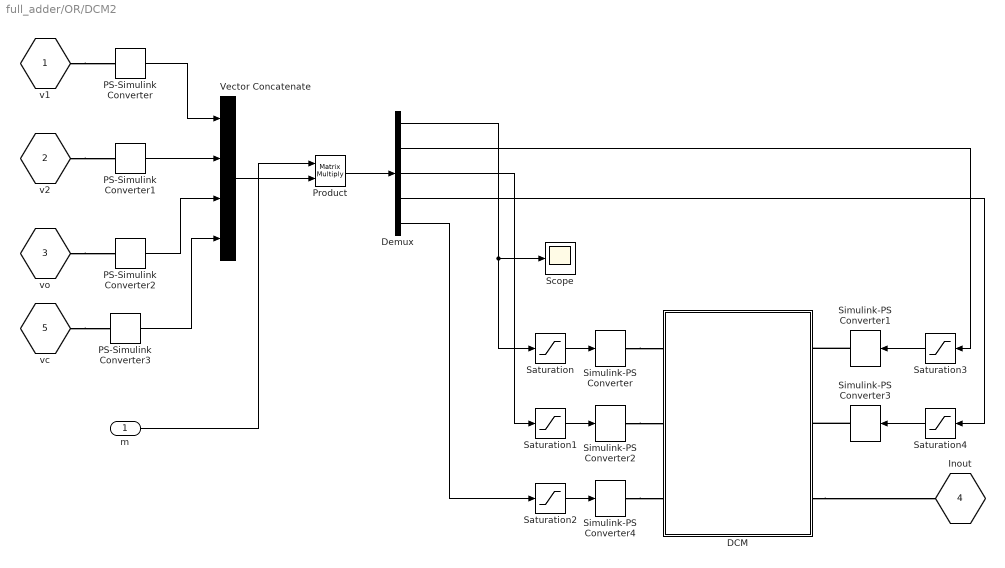
== system full_adder/OR/DCM2 ==
  m : Inport
  DCM : Subsystem
  Demux : Demux  Outputs=5
  PS-Simulink Converter{,1..3} (4 alike) : nesl_utility/PS-Simulink Converter  PhysicalDomain=network_engine_domain  SubClassName=ps_output  LeftPortType=input  RightPortType=output  PseudoPeriodic=off  Frequencies=[]  Unit=V  AffineConversion=off
  Product : Product  Multiplication=Matrix(*)
  Saturation{,1..4} (5 alike) : Saturate  UpperLimit=10  LowerLimit=-10
  Scope : Scope
      settings: YMin=-30  YMax=15  SaveName=ScopeData3
  Simulink-PS Converter{,1..4} (5 alike) : nesl_utility/Simulink-PS Converter  PhysicalDomain=network_engine_domain  SubClassName=ps_input  LeftPortType=input  RightPortType=output  PseudoPeriodic=off  Frequencies=[]  NoiseDistribution=none  NoiseParameters=[]  Unit=V  AffineConversion=off  InputFiltering=off  SimscapeFilterOrder=1  InputFilterTimeConstant=0.001  UdotUserProvided=1
  Vector Concatenate : Concatenate  NumInputs=4
  "v1 " : PMIOPort  Port=1  Side=Left
  v2 : PMIOPort  Port=2  Side=Right
  vo : PMIOPort  Port=3  Side=Left
  Inout : PMIOPort  Port=4  Side=Right
  vc : PMIOPort  Port=5  Side=Left
  wires:
  PS-Simulink Converter3/1 -> Vector Concatenate/4
  PS-Simulink Converter/1 -> Vector Concatenate/1
  PS-Simulink Converter2/1 -> Vector Concatenate/3
  PS-Simulink Converter1/1 -> Vector Concatenate/2
  Demux/1 -> Scope/1, Saturation/1
  m/1 -> Product/1
  Vector Concatenate/1 -> Product/2
  Product/1 -> Demux/1
  Saturation/1 -> Simulink-PS Converter/1
  Demux/3 -> Saturation1/1
  Saturation1/1 -> Simulink-PS Converter2/1
  Demux/5 -> Saturation2/1
  Saturation2/1 -> Simulink-PS Converter4/1
  Saturation3/1 -> Simulink-PS Converter1/1
  Demux/2 -> Saturation3/1
  Saturation4/1 -> Simulink-PS Converter3/1
  Demux/4 -> Saturation4/1
  connections:
  Simulink-PS Converter2/RConn1 -- DCM/LConn2
  DCM/RConn3 -- Inout/RConn1
  Simulink-PS Converter3/RConn1 -- DCM/RConn2
  vo/RConn1 -- PS-Simulink Converter2/LConn1
  Simulink-PS Converter4/RConn1 -- DCM/LConn3
  Simulink-PS Converter/RConn1 -- DCM/LConn1
  "v1 "/RConn1 -- PS-Simulink Converter/LConn1
  v2/RConn1 -- PS-Simulink Converter1/LConn1
  Simulink-PS Converter1/RConn1 -- DCM/RConn1
  vc/RConn1 -- PS-Simulink Converter3/LConn1

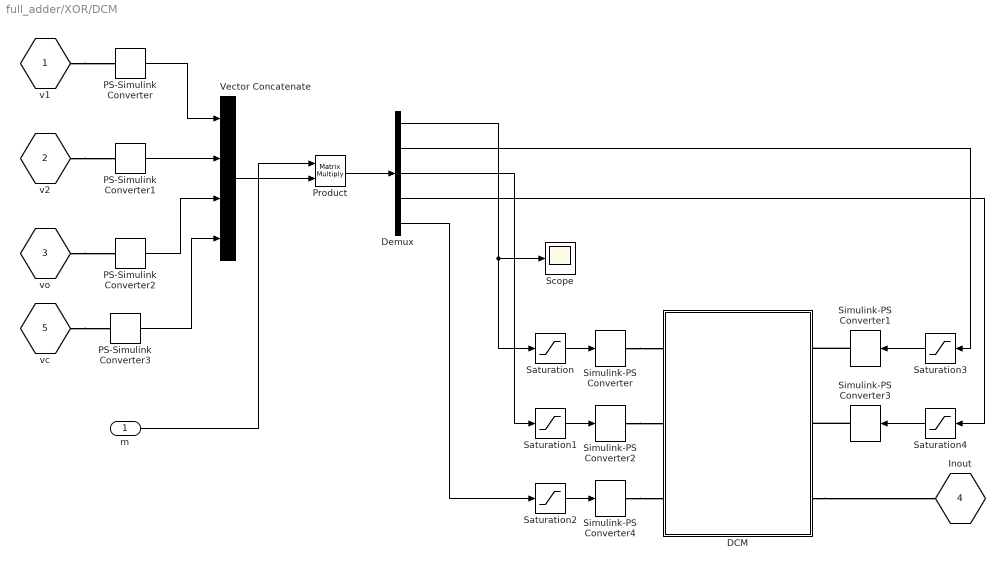
== system full_adder/XOR/DCM ==
  m : Inport
  DCM : Subsystem
  Demux : Demux  Outputs=5
  PS-Simulink Converter{,1..3} (4 alike) : nesl_utility/PS-Simulink Converter  PhysicalDomain=network_engine_domain  SubClassName=ps_output  LeftPortType=input  RightPortType=output  PseudoPeriodic=off  Frequencies=[]  Unit=V  AffineConversion=off
  Product : Product  Multiplication=Matrix(*)
  Saturation{,1..4} (5 alike) : Saturate  UpperLimit=10  LowerLimit=-10
  Scope : Scope
      settings: YMin=-30  YMax=15  SaveName=ScopeData3
  Simulink-PS Converter{,1..4} (5 alike) : nesl_utility/Simulink-PS Converter  PhysicalDomain=network_engine_domain  SubClassName=ps_input  LeftPortType=input  RightPortType=output  PseudoPeriodic=off  Frequencies=[]  NoiseDistribution=none  NoiseParameters=[]  Unit=V  AffineConversion=off  InputFiltering=off  SimscapeFilterOrder=1  InputFilterTimeConstant=0.001  UdotUserProvided=1
  Vector Concatenate : Concatenate  NumInputs=4
  "v1 " : PMIOPort  Port=1  Side=Left
  v2 : PMIOPort  Port=2  Side=Right
  vo : PMIOPort  Port=3  Side=Left
  Inout : PMIOPort  Port=4  Side=Right
  vc : PMIOPort  Port=5  Side=Left
  wires:
  PS-Simulink Converter3/1 -> Vector Concatenate/4
  PS-Simulink Converter/1 -> Vector Concatenate/1
  PS-Simulink Converter2/1 -> Vector Concatenate/3
  PS-Simulink Converter1/1 -> Vector Concatenate/2
  Demux/1 -> Scope/1, Saturation/1
  m/1 -> Product/1
  Vector Concatenate/1 -> Product/2
  Product/1 -> Demux/1
  Saturation/1 -> Simulink-PS Converter/1
  Demux/3 -> Saturation1/1
  Saturation1/1 -> Simulink-PS Converter2/1
  Demux/5 -> Saturation2/1
  Saturation2/1 -> Simulink-PS Converter4/1
  Saturation3/1 -> Simulink-PS Converter1/1
  Demux/2 -> Saturation3/1
  Saturation4/1 -> Simulink-PS Converter3/1
  Demux/4 -> Saturation4/1
  connections:
  Simulink-PS Converter2/RConn1 -- DCM/LConn2
  DCM/RConn3 -- Inout/RConn1
  Simulink-PS Converter3/RConn1 -- DCM/RConn2
  vo/RConn1 -- PS-Simulink Converter2/LConn1
  Simulink-PS Converter4/RConn1 -- DCM/LConn3
  Simulink-PS Converter/RConn1 -- DCM/LConn1
  "v1 "/RConn1 -- PS-Simulink Converter/LConn1
  v2/RConn1 -- PS-Simulink Converter1/LConn1
  Simulink-PS Converter1/RConn1 -- DCM/RConn1
  vc/RConn1 -- PS-Simulink Converter3/LConn1

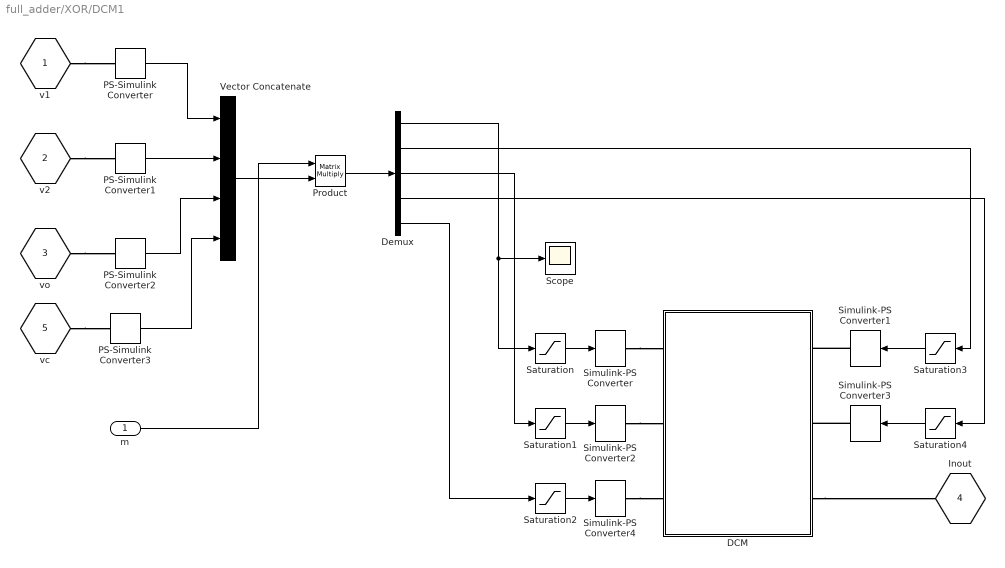
== system full_adder/XOR/DCM1 ==
  m : Inport
  DCM : Subsystem
  Demux : Demux  Outputs=5
  PS-Simulink Converter{,1..3} (4 alike) : nesl_utility/PS-Simulink Converter  PhysicalDomain=network_engine_domain  SubClassName=ps_output  LeftPortType=input  RightPortType=output  PseudoPeriodic=off  Frequencies=[]  Unit=V  AffineConversion=off
  Product : Product  Multiplication=Matrix(*)
  Saturation{,1..4} (5 alike) : Saturate  UpperLimit=10  LowerLimit=-10
  Scope : Scope
      settings: YMin=-30  YMax=15  SaveName=ScopeData3
  Simulink-PS Converter{,1..4} (5 alike) : nesl_utility/Simulink-PS Converter  PhysicalDomain=network_engine_domain  SubClassName=ps_input  LeftPortType=input  RightPortType=output  PseudoPeriodic=off  Frequencies=[]  NoiseDistribution=none  NoiseParameters=[]  Unit=V  AffineConversion=off  InputFiltering=off  SimscapeFilterOrder=1  InputFilterTimeConstant=0.001  UdotUserProvided=1
  Vector Concatenate : Concatenate  NumInputs=4
  "v1 " : PMIOPort  Port=1  Side=Left
  v2 : PMIOPort  Port=2  Side=Right
  vo : PMIOPort  Port=3  Side=Left
  Inout : PMIOPort  Port=4  Side=Right
  vc : PMIOPort  Port=5  Side=Left
  wires:
  PS-Simulink Converter3/1 -> Vector Concatenate/4
  PS-Simulink Converter/1 -> Vector Concatenate/1
  PS-Simulink Converter2/1 -> Vector Concatenate/3
  PS-Simulink Converter1/1 -> Vector Concatenate/2
  Demux/1 -> Scope/1, Saturation/1
  m/1 -> Product/1
  Vector Concatenate/1 -> Product/2
  Product/1 -> Demux/1
  Saturation/1 -> Simulink-PS Converter/1
  Demux/3 -> Saturation1/1
  Saturation1/1 -> Simulink-PS Converter2/1
  Demux/5 -> Saturation2/1
  Saturation2/1 -> Simulink-PS Converter4/1
  Saturation3/1 -> Simulink-PS Converter1/1
  Demux/2 -> Saturation3/1
  Saturation4/1 -> Simulink-PS Converter3/1
  Demux/4 -> Saturation4/1
  connections:
  Simulink-PS Converter2/RConn1 -- DCM/LConn2
  DCM/RConn3 -- Inout/RConn1
  Simulink-PS Converter3/RConn1 -- DCM/RConn2
  vo/RConn1 -- PS-Simulink Converter2/LConn1
  Simulink-PS Converter4/RConn1 -- DCM/LConn3
  Simulink-PS Converter/RConn1 -- DCM/LConn1
  "v1 "/RConn1 -- PS-Simulink Converter/LConn1
  v2/RConn1 -- PS-Simulink Converter1/LConn1
  Simulink-PS Converter1/RConn1 -- DCM/RConn1
  vc/RConn1 -- PS-Simulink Converter3/LConn1

== system full_adder/XOR/DCM2 ==
  m : Inport
  DCM : Subsystem
  Demux : Demux  Outputs=5
  PS-Simulink Converter{,1..3} (4 alike) : nesl_utility/PS-Simulink Converter  PhysicalDomain=network_engine_domain  SubClassName=ps_output  LeftPortType=input  RightPortType=output  PseudoPeriodic=off  Frequencies=[]  Unit=V  AffineConversion=off
  Product : Product  Multiplication=Matrix(*)
  Saturation{,1..4} (5 alike) : Saturate  UpperLimit=10  LowerLimit=-10
  Scope : Scope
      settings: YMin=-30  YMax=15  SaveName=ScopeData3
  Simulink-PS Converter{,1..4} (5 alike) : nesl_utility/Simulink-PS Converter  PhysicalDomain=network_engine_domain  SubClassName=ps_input  LeftPortType=input  RightPortType=output  PseudoPeriodic=off  Frequencies=[]  NoiseDistribution=none  NoiseParameters=[]  Unit=V  AffineConversion=off  InputFiltering=off  SimscapeFilterOrder=1  InputFilterTimeConstant=0.001  UdotUserProvided=1
  Vector Concatenate : Concatenate  NumInputs=4
  "v1 " : PMIOPort  Port=1  Side=Left
  v2 : PMIOPort  Port=2  Side=Right
  vo : PMIOPort  Port=3  Side=Left
  Inout : PMIOPort  Port=4  Side=Right
  vc : PMIOPort  Port=5  Side=Left
  wires:
  PS-Simulink Converter3/1 -> Vector Concatenate/4
  PS-Simulink Converter/1 -> Vector Concatenate/1
  PS-Simulink Converter2/1 -> Vector Concatenate/3
  PS-Simulink Converter1/1 -> Vector Concatenate/2
  Demux/1 -> Scope/1, Saturation/1
  m/1 -> Product/1
  Vector Concatenate/1 -> Product/2
  Product/1 -> Demux/1
  Saturation/1 -> Simulink-PS Converter/1
  Demux/3 -> Saturation1/1
  Saturation1/1 -> Simulink-PS Converter2/1
  Demux/5 -> Saturation2/1
  Saturation2/1 -> Simulink-PS Converter4/1
  Saturation3/1 -> Simulink-PS Converter1/1
  Demux/2 -> Saturation3/1
  Saturation4/1 -> Simulink-PS Converter3/1
  Demux/4 -> Saturation4/1
  connections:
  Simulink-PS Converter2/RConn1 -- DCM/LConn2
  DCM/RConn3 -- Inout/RConn1
  Simulink-PS Converter3/RConn1 -- DCM/RConn2
  vo/RConn1 -- PS-Simulink Converter2/LConn1
  Simulink-PS Converter4/RConn1 -- DCM/LConn3
  Simulink-PS Converter/RConn1 -- DCM/LConn1
  "v1 "/RConn1 -- PS-Simulink Converter/LConn1
  v2/RConn1 -- PS-Simulink Converter1/LConn1
  Simulink-PS Converter1/RConn1 -- DCM/RConn1
  vc/RConn1 -- PS-Simulink Converter3/LConn1
